simulink model "FinalVersion+AdaptiveSpeedModulation"  (R2024b)
settings: Solver=FixedStepAuto  StartTime=0.0  StopTime=inf  FixedStep=0.001  RelTol=1e-3  EnableMultiTasking=on
libraries: dspnetwork x7
settings Model: xpc_rtwmakecfg_data=_xpcnblib__xpcetherlib__xpcether8255xlib__xpcetherGbElib__xpciplib_  Creator=rudol  LastModifiedBy=Sanjay
settings SolverCC: AlgebraicLoopSolver=TrustRegion
settings DataIOCC: LimitDataPoints=on  SaveFormat=Array  ReturnWorkspaceOutputs=off
settings OptimizationCC: ReuseModelBlockBuffer=off  LifeSpan=inf
settings DebuggingCC: UnconnectedInputMsg=warning  UnconnectedOutputMsg=warning  UnconnectedLineMsg=warning  SFUnexpectedBacktrackingDiag=warning  SFNoUnconditionalDefaultTransitionDiag=warning  SFExecutionAtInitializationDiag=none  ArithmeticOperatorsInVariantConditions=warning
settings HardwareCC: ProdBitPerPointer=32  ProdBitPerSizeT=32  ProdBitPerPtrDiffT=32  ProdLargestAtomicFloat=None  ProdIntDivRoundTo=Undefined  ProdEndianess=Unspecified  ProdWordSize=32  ProdHWDeviceType=32-bit Generic
settings ModelReferenceCC: PropagateSignalLabelsOutOfModel=off
settings SFSimCC: SimUseLocalCustomCode=off  CustomCodeUndefinedFunction=UseInterfaceOnly
settings RTWCC: RTWUseLocalCustomCode=off  GPUComputeCapability=3.5
settings CodeAppCC: StateflowObjectComments=on
settings GRTTargetCC: TargetLangStandard=C89/C90 (ANSI)
settings ConfigComp: CovMetricSettings=dw  CovSaveCumulativeToWorkspaceVar=on  CovSaveSingleToWorkspaceVar=on  CovExternalEMLEnable=off

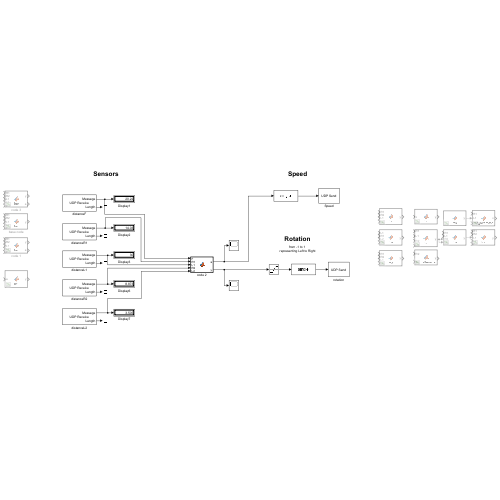
[thumbnail: Simulink's stored preview of the top-level diagram]
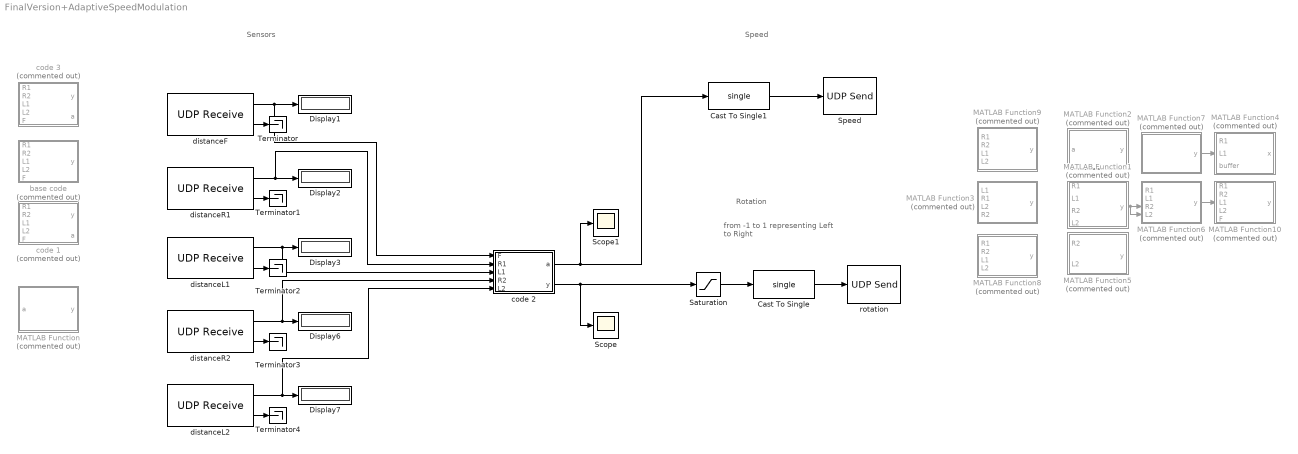
== system FinalVersion+AdaptiveSpeedModulation ==
  note: Sensors
  note: from -1 to 1
      | representing Left to Right
  note: Speed
  note: Rotation
  Cast To Single : DataTypeConversion  OutDataTypeStr=single  SaturateOnIntegerOverflow=off  RndMeth=Floor
  Cast To Single1 : DataTypeConversion  OutDataTypeStr=single  SaturateOnIntegerOverflow=off  RndMeth=Floor
  Display{1..3,6..7} (5 alike) : Display
  MATLAB Function : MATLAB Function  Commented=on  TreatAsAtomicUnit=on
  MATLAB Function1 : MATLAB Function  Commented=on  TreatAsAtomicUnit=on
  MATLAB Function10 : MATLAB Function  Commented=on  TreatAsAtomicUnit=on
  MATLAB Function2 : MATLAB Function  Commented=on  TreatAsAtomicUnit=on
  MATLAB Function3 : MATLAB Function  Commented=on  TreatAsAtomicUnit=on
  MATLAB Function4 : MATLAB Function  Commented=on  TreatAsAtomicUnit=on
  MATLAB Function5 : MATLAB Function  Commented=on  TreatAsAtomicUnit=on
  MATLAB Function6 : MATLAB Function  Commented=on  TreatAsAtomicUnit=on
  MATLAB Function7 : MATLAB Function  Commented=on  TreatAsAtomicUnit=on
  MATLAB Function8 : MATLAB Function  Commented=on  TreatAsAtomicUnit=on
  MATLAB Function9 : MATLAB Function  Commented=on  TreatAsAtomicUnit=on
  Saturation : Saturate  UpperLimit=1  LowerLimit=-1
  Scope : Scope
  Scope1 : Scope
  Speed : dspnetwork/UDP Send  remoteURL='127.0.0.1'  remotePort=55501  localURL='0.0.0.0'  localPortSource=Automatically determine  localPort=-1  sendBufferSize=8192  sampletime=-1  blockPlatform=[]  separateLengthPort=0
  Terminator{,1..4} (5 alike) : Terminator
  base code : MATLAB Function  Commented=on  TreatAsAtomicUnit=on
  code 1 : MATLAB Function  Commented=on  TreatAsAtomicUnit=on
  code 2 : MATLAB Function  TreatAsAtomicUnit=on
  code 3 : MATLAB Function  Commented=on  TreatAsAtomicUnit=on
  distanceF : dspnetwork/UDP Receive  localURL='0.0.0.0'  localPort=10  remoteURL='0.0.0.0'  remotePort=-1  recvBufferSize=8192  dims=1  signalDatatype=single  isComplex=off  isVarSize=off  showBlockingTime=off  blockingTime=0  sampletime=0.001  blockPlatform=[]
  distanceL1 : dspnetwork/UDP Receive  localURL='0.0.0.0'  localPort=12  remoteURL='0.0.0.0'  remotePort=-1  recvBufferSize=8192  dims=1  signalDatatype=single  isComplex=off  isVarSize=off  showBlockingTime=off  blockingTime=0  sampletime=0.001  blockPlatform=[]
  distanceL2 : dspnetwork/UDP Receive  localURL='0.0.0.0'  localPort=14  remoteURL='0.0.0.0'  remotePort=-1  recvBufferSize=8192  dims=1  signalDatatype=single  isComplex=off  isVarSize=off  showBlockingTime=off  blockingTime=0  sampletime=0.001  blockPlatform=[]
  distanceR1 : dspnetwork/UDP Receive  localURL='0.0.0.0'  localPort=11  remoteURL='0.0.0.0'  remotePort=-1  recvBufferSize=8192  dims=1  signalDatatype=single  isComplex=off  isVarSize=off  showBlockingTime=off  blockingTime=0  sampletime=0.001  blockPlatform=[]
  distanceR2 : dspnetwork/UDP Receive  localURL='0.0.0.0'  localPort=13  remoteURL='0.0.0.0'  remotePort=-1  recvBufferSize=8192  dims=1  signalDatatype=single  isComplex=off  isVarSize=off  showBlockingTime=off  blockingTime=0  sampletime=0.001  blockPlatform=[]
  rotation : dspnetwork/UDP Send  remoteURL='127.0.0.1'  remotePort=55000  localURL='0.0.0.0'  localPortSource=Automatically determine  localPort=-1  sendBufferSize=8192  sampletime=-1  blockPlatform=[]  separateLengthPort=0
  wires:
  distanceL1/1 -> Display3/1, code 2/3(L1)
  distanceR1/1 -> code 2/2(R1), Display2/1
  distanceR2/1 -> Display6/1, code 2/4(R2)
  distanceL2/1 -> code 2/5(L2), Display7/1
  Cast To Single/1 -> rotation/1
  distanceF/1 -> Display1/1, code 2/1(F)
  distanceF/2 -> Terminator/1
  distanceR1/2 -> Terminator1/1
  distanceL1/2 -> Terminator2/1
  distanceR2/2 -> Terminator3/1
  distanceL2/2 -> Terminator4/1
  Saturation/1 -> Cast To Single/1
  Cast To Single1/1 -> Speed/1
  code 2/1(a) -> Scope1/1, Cast To Single1/1
  MATLAB Function7/1(y) -> MATLAB Function4/2(L1)
  MATLAB Function1/1(y) -> MATLAB Function6/4(L2), MATLAB Function6/3(R2)
  MATLAB Function6/1(y) -> MATLAB Function10/3(L1)
  code 2/2(y) -> Scope/1, Saturation/1

== matlab function FinalVersion+AdaptiveSpeedModulation/MATLAB Function10 ==
  data: R1 input; y output; R2 input; L1 input; L2 input; F input
function y = fnc(R1, R2, L1, L2, F)
    % Ensure all inputs are of type double to avoid type mismatch
    R1 = double(R1);
    R2 = double(R2);
    L1 = double(L1);
    L2 = double(L2);
    F = double(F);
    y = 0;
    
    % Calculate averages for turning behavior
    avg_RF = (R1 + F) / 2; 
    avg_FL = (F + L1) / 2;   
    avg_R2L2 = (R2 + L2) / 2;  

    % Speed adjustment based on proximity to obstacles
    if R1 < 5 || R2 < 5
        y = -0.7;  
        if R1 < 2.5 || R2 < 2.5
            y = -1;  
        end
    elseif L1 < 5 || L2 < 5
        y = 0.7; 
        if L1 < 5 / 2 || L2 < 5 / 2
            y = 1; 
        end
    end

    % Right turn behavior using front and right-side sensors (smooth turning)
    if avg_RF < 5
        
        y = -1* (5 - avg_RF) ;  
    end

    % Left turn behavior using front and left-side sensors (smooth turning)
    if avg_FL < 5
        
        y =   (5 - avg_FL) ; 
    end

    % Keep the car centered using R2 and L2 (center alignment logic)
    if abs(R2 - L2) > 2.5 
        
        if R2 > L2
            y = y + (R2 - L2) ; 
        elseif L2 > R2
            y = y - (L2 - R2) ; 
        end
    end
    % Additional fine-tuning for smoother operation
    if abs(R2 - L2) < 2.5
        y = y * 0.5;  
    end
end

== matlab function FinalVersion+AdaptiveSpeedModulation/code 1 ==
  data: R1 input; y output; R2 input; L1 input; L2 input; F input; a output
function [y, a] = fnc(R1, R2, L1, L2, F)
    % Ensure all inputs are of type double to avoid type mismatch
    R1 = double(R1);
    R2 = double(R2);
    L1 = double(L1);
    L2 = double(L2);
    F = double(F);
    a = double(F);
    y = 0;  % Steering adjustment
    safe_distance = 5;  % Default safe distance threshold for obstacle avoidance
    
    % Calculate averages for turning behavior
    avg_RF = (R1 + F) / 2;  % Average of Front sensor and Right side sensor
    avg_FL = (F + L1) / 2;  % Average of Front sensor and Left side sensor
    avg_R2L2 = (R2 + L2) / 2;  % Average of Back Right and Back Left sensors (for track center)
    avg_R1L1 = (R1 + L1) / 2;  % Average of Right and Left side sensors (for track center)
     if a < 10
        a = a - (0.2 * F);  % Gradual slowdown based on front sensor proximity
    else
        a = 4 * F;  % Keep a stable speed if the distance is far enough
    end
    
    % Reduce safe distance in the corner (turning condition)
    if abs(avg_RF - avg_FL) > 2  % Corner detected when there is a significant difference in sensor readings
        safe_distance = 3;  % Reduce safe distance during sharp turns
    end
    
    % Speed adjustment based on proximity to obstacles
    if R1 < safe_distance || R2 < safe_distance
        % Slow down if too close to the right side
        y = -5;  % Turn slightly left
        a = 3 * F;  % Reduce speed
        if R1 < safe_distance / 2 || R2 < safe_distance / 2
            y = -10;  % Slow down more if dangerously close to the right side
            a = 2 * F;  % Further reduce speed
        end
    elseif L1 < safe_distance || L2 < safe_distance
        % Speed up if approaching the left side
        y = 5;  % Turn slightly right
        a = 3 * F;  % Increase speed a bit
        if L1 < safe_distance / 2 || L2 < safe_distance / 2
            y = 10;  % Speed up more if dangerously close to the left side
            a = 4 * F;  % Increase speed further
        end
    end
    
    % Smooth turning behavior based on the proximity of the front sensors
    if avg_RF < 3  % Right turn behavior
        y = -5 * (15 - avg_RF) / 15;  % Smooth turning to the right (gradual turn)
        a = 3 * F;  % Maintain speed
    elseif avg_FL < 3  % Left turn behavior
        y = 5 * (15 - avg_FL) / 15;  % Smooth turning to the left (gradual turn)
        a = 3 * F;  % Maintain speed
    end
    
    % Keep the car centered using R2 and L2 (center alignment logic)
    if abs(R2 - L2) > safe_distance / 2  % Check if the car is off-center
        % Apply dynamic steering based on how far off-center the car is
        if R2 > L2
            y = y + 5 * (R2 - L2) / safe_distance;  % Turn left to bring the car back to the center
        elseif L2 > R2
            y = y - 5 * (L2 - R2) / safe_distance;  % Turn right to bring the car back to the center
        end
    end
    
    % % Keep the car centered using R1 and L1 (center alignment logic)
    % if abs(R1 - L1) > safe_distance / 2  % Check if the car is off-center
    %     % Apply dynamic steering based on how far off-center the car is
    %     if R1 > L1
    %         y = y + 5 * (R1 - L1) / safe_distance;  % Turn left to bring the car back to the center
    %     elseif L1 > R1
    %         y = y - 5 * (L1 - R1) / safe_distance;  % Turn right to bring the car back to the center
    %     end
    % end
    
    % Smooth out steering behavior when the rear sensors are close
    if abs(R2 - L2) < safe_distance / 3
        y = y * 0.5;  % Reduce steering to make it smoother when the car is near the center
    end
    
    % High-speed cornering logic (when speed is high and sensors indicate a turn)
    if F > 50 && (avg_RF < safe_distance || avg_FL < safe_distance)
        % Increase turn speed and make it sharper
        if avg_RF < avg_FL
            y = -20;  % Turn right aggressively during sharp turn
            a = 6 * F;  % Maintain higher speed for sharp turn
        else
            y = 20;  % Turn left aggressively during sharp turn
            a = 6 * F;  % Maintain higher speed for sharp turn
        end
    end
    
    % Return the computed steering and acceleration values
end

== matlab function FinalVersion+AdaptiveSpeedModulation/base code ==
  data: R1 input; y output; R2 input; L1 input; L2 input; F input
function y = fnc(R1, R2, L1, L2, F)
    % Ensure all inputs are of type double to avoid type mismatch
    R1 = double(R1);
    R2 = double(R2);
    L1 = double(L1);
    L2 = double(L2);
    F = double(F);
    
    y = 0;
    safe_distance = 5;

    % Calculate averages for turning behavior
    avg_RF = (R1 + F) / 2;  % Average of Front sensor and Right side sensor
    avg_FL = (F + L1) / 2;   % Average of Front sensor and Left side sensor
    avg_R2L2 = (R2 + L2) / 2;  % Average of Back Right and Back Left sensors (for track center)

    % Speed adjustment based on proximity to obstacles
    if R1 < safe_distance || R2 < safe_distance
        y = -10;  % Slow down if too close to the right side
        if R1 < safe_distance / 2 || R2 < safe_distance / 2
            y = -15;  % Slow down more if dangerously close to the right side
        end
    elseif L1 < safe_distance || L2 < safe_distance
        y = 10;  % Speed up if approaching left side
        if L1 < safe_distance / 2 || L2 < safe_distance / 2
            y = 15;  % Speed up more if dangerously close to the left side
        end
    end

    % High-speed turning decision (based on front sensors)
    if (R1 < safe_distance || R2 < safe_distance) && (L1 < safe_distance || L2 < safe_distance)
        if min(R1, R2) > min(L1, L2)
            y = 10;  % Likely turning right, increase right steering
        else
            y = -10;  % Likely turning left, increase left steering
        end
    end

    % Right turn behavior using front and right-side sensors (smooth turning)
    if avg_RF < safe_distance
        % Smooth turning to the right (gradual turn)
        y = -5 * (safe_distance - avg_RF) / safe_distance;  % Adjust turning intensity based on proximity
    end

    % Left turn behavior using front and left-side sensors (smooth turning)
    if avg_FL < safe_distance
        % Smooth turning to the left (gradual turn)
        y = 5 * (safe_distance - avg_FL) / safe_distance;  % Adjust turning intensity based on proximity
    end

    % Keep the car centered using R2 and L2 (center alignment logic)
    if abs(R2 - L2) > safe_distance / 2  % Check if car is off-center
        % Apply a dynamic steering based on how far off-center the car is
        if R2 > L2
            y = y + 5 * (R2 - L2) / safe_distance;  % Turn left to bring the car back to the center
        elseif L2 > R2
            y = y - 5 * (L2 - R2) / safe_distance;  % Turn right to bring the car back to the center
        end
    end

    % Additional fine-tuning for smoother operation
    % If the difference between rear sensors is small, don't apply harsh steering
    if abs(R2 - L2) < safe_distance / 3
        y = y * 0.5;  % Reduce steering to make it smoother when the car is near center
    end
end

== matlab function FinalVersion+AdaptiveSpeedModulation/code 3 ==
  data: R1 input; y output; R2 input; L1 input; L2 input; F input; a output
function [y,a] = fnc(R1, R2, L1, L2, F)
    % Ensure all inputs are of type double to avoid type mismatch
    R1 = double(R1);
    R2 = double(R2);
    L1 = double(L1);
    L2 = double(L2);
    F = double(F);
    a=double(F);
    y = 0;
    safe_distance = 5;
    
    % Calculate averages for turning behavior
    avg_RF = (R1 + F) / 2; % Average of Front sensor and Right side sensor
    avg_FL = (F + L1) / 2; % Average of Front sensor and Left side sensor
    avg_R2L2 = (R2 + L2) / 2; % Average of Back Right and Back Left sensors (for track center)
    avg_R1L1 = (R1 + L1) / 2; % Average of Right and Left side sensors (for track center)
     if a < 10
        a = a -(0.2* F);  
    else
        a = 4*F;  
    end
    
    % Speed adjustment based on proximity to obstacles
    if R1 < safe_distance || R2 < safe_distance
        y = -10; % Slow down if too close to the right side
        a=4*F;
        if R1 < safe_distance / 2 || R2 < safe_distance / 2
            y = -15; % Slow down more if dangerously close to the right side
            a=3.5*F;
        end
    elseif L1 < safe_distance || L2 < safe_distance
        y = 10; % Speed up if approaching left side
        a=4*F;
        if L1 < safe_distance / 2 || L2 < safe_distance / 2
            y = 15; % Speed up more if dangerously close to the left side
            a=3.5*F;
        end
    end
    
    % High-speed turning decision (based on front sensors)
    if (R1 < safe_distance || R2 < safe_distance) && (L1 < safe_distance || L2 < safe_distance)
        if min(R1, R2) > min(L1, L2)
            y = 10; % Likely turning right, increase right steering
            a=4*F;
        else
            y = -10; % Likely turning left, increase left steering
            a=6*F;
        end
    end
    
    % Right turn behavior using front and right-side sensors (smooth turning)
    if avg_RF < 3
        % Smooth turning to the right (gradual turn)
        y = -5 * (15 - avg_RF) / 15; % Adjust turning intensity based on proximity
        a=4.5*F;
    end
    
    % Left turn behavior using front and left-side sensors (smooth turning)
    if avg_FL < 3
        % Smooth turning to the left (gradual turn)
        y = 5 * (15 - avg_FL) / 15; % Adjust turning intensity based on proximity
        a=4.5*F;
    end
    
    % Keep the car centered using R2 and L2 (center alignment logic)
    if abs(R2 - L2) > safe_distance / 2
        % Check if car is off-center
        % Apply a dynamic steering based on how far off-center the car is
        if R2 > L2
            y = y + 5 * (R2 - L2) / safe_distance; % Turn left to bring the car back to the center
        elseif L2 > R2
            y = y - 5 * (L2 - R2) / safe_distance; % Turn right to bring the car back to the center
        end
    end
    
    % Keep the car centered using R1 and L1 (center alignment logic)
    if abs(R1 - L1) > safe_distance / 2
        % Check if car is off-center
        % Apply a dynamic steering based on how far off-center the car is
        if R1 > L1
            y = y + 5 * (R1 - L1) / safe_distance; % Turn left to bring the car back to the center
        elseif L1 > R1
            y = y - 5 * (L1 - R1) / safe_distance; % Turn right to bring the car back to the center
        end
    end
    
    % Additional fine-tuning for smoother operation
    % If the difference between rear sensors is small, don't apply harsh steering
    if abs(R2 - L2) < safe_distance / 3
        y = y * 0.5; % Reduce steering to make it smoother when the car is near center
    end
    
    % High-speed cornering logic
    if F > 50 && (avg_RF < safe_distance || avg_FL < safe_distance)
        if avg_RF < avg_FL
            y = -15; % Turn right sharply
            a=4*F;
        else
            y = 15; % Turn left sharply
            a=4*F;
        end
    end
end

== matlab function FinalVersion+AdaptiveSpeedModulation/code 2 ==
  data: F input; a output; R1 input; L1 input; y output; R2 input; L2 input
function [a, y] = fnc(F,R1, L1, R2, L2)
    R1 = double(R1);
    R2 = double(R2);
    L1 = double(L1);
    L2 = double(L2);
    F = double(F);
    a = double(F);
    y = 0;  
     
    avg_RF = (R1 + F) / 2;  
    avg_FL = (F + L1) / 2;  
    avg_R2L2 = (R2 + L2) / 2;  % this function not used in logic 
    avg_R1L1 = (R1 + L1) / 2;  % this function not used in logic 
    
    if a < 10        
        a = a - (0.2 * F);  % I reduced the car speed gradually based on front sensor proximity
    else
        a = 4.5* F; 
   end    
    
   %buffer zone =5;
    
   if R1 < 5 || R2 < 5               
        y = -0.5;   % turn left slightly based on if condition
        a = 3 * F; 
       
        %buffer zone =5;
        %(buffer zone/2)=2.5;
        if R1 < 2.5 || R2 < 2.5
            y = -1;  % it will turn left suddenly
            a = 4 * F;  
        end
        
        %buffer zone =5;
    elseif L1 < 5 || L2 < 5
        
        y = 0.5;  % Turn slightly right
        a = 3 * F;  
        
        %buffer zone =5;
        %(buffer zone/2)=2.5;
        if L1 < 2.5|| L2 < 2.5
            y = 1;  % it will rurn right suddenly
            a = 4 * F; 
        end
    end
    
    if avg_RF < 3 
        y = -5 * (15 - avg_RF) / 15;  %gradual turn
        a = 3 * F;  
    elseif avg_FL < 3 
        y = 5 * (15 - avg_FL) / 15;  % gradual turn
        a = 3 * F;  
    end

    %buffer zone =3; (buffer zone / 2)=1.5;
    if abs(R2 - L2) >1.5  % Check if the car is off-center  
        
        if R2 > L2
            y = y + 5 * (R2 - L2) / 3;  % Turn left to bring the car back to the center
        elseif L2 > R2
            y = y - 5 * (L2 - R2) / 3;  % Turn right to bring the car back to the center
        end
    end
    
    %buffer zone =3; (buffer zone / 2)=1.5;
    if abs(R1 - L1) > 1.5  % Check if the car is off-center
        if R1 > L1
            y = y + 5 * (R1 - L1) / 3;  % Turn left to bring the car back to the center
        elseif L1 > R1
            y = y - 5 * (L1 - R1) / 3;  % Turn right to bring the car back to the center
        end
    end
    
   %buffer zone =5;
    if abs(R2 - L2) < 5 / 3
        y = y * 0.5;  % Reduce steering to make it smoother when the car is near the center
    end
    
    %buffer zone = 5;
    if F > 50 && (avg_RF < 5 || avg_FL < 5)   %  when speed is high and sensors indicate a turn
        if avg_RF < avg_FL
            y = -15;  % Turn right sharply
            a = 4 * F;  
        else
            y = 15;  % Turn left sharply
            a = 4 * F;  
        end
    end
end

== matlab function FinalVersion+AdaptiveSpeedModulation/MATLAB Function1 ==
  data: R1 input; L1 input; R2 input; y output; L2 input
function y = fcn(R1, L1,R2,L2)
  Kp = 1.5;
    left_distance = (L1 + L2) / 2;
    right_distance = (R1 + R2) / 2;
    error = left_distance - right_distance;
    y = -Kp * error;
    safe_distance = 20; 
    max_steering_angle = 30; 

    if R1 < safe_distance
        right_adjustment = max_steering_angle * (safe_distance - R1) / safe_distance;
        y = y + right_adjustment;
    end
     
    if L1 < safe_distance
        left_adjustment = max_steering_angle * (safe_distance - L1) / safe_distance;
        y = y - left_adjustment;
    end
    if R2 < safe_distance
        right_adjustment = max_steering_angle * (safe_distance - R2) / safe_distance;
        y = y + right_adjustment * 0.5;
    end

    if L2 < safe_distance
        left_adjustment = max_steering_angle * (safe_distance - L2) / safe_distance;
        y = y - left_adjustment * 0.5;
    end
 y = max(min(y, max_steering_angle), -max_steering_angle);

   
end

== matlab function FinalVersion+AdaptiveSpeedModulation/MATLAB Function ==
  data: a input; y output
function y = fcn(a)    
    
    if a < 10
        a = a -(0.2* a);  
    else
        a = a + (4.5* a);  
    end
  
y=a;
end



  % a: current speed
    % curvature: turn's curvature (higher value means tighter turn)

    %if curvature > 0.5
        % Tight turn, reduce speed
        %a = a - (0.2 * a);
    %elseif curvature < -0.5
        % Tight turn, reduce speed
       % a = a - (0.2 * a);
   % else
        % Smooth turn or straight path, maintain or increase speed
       % a = a + (0.1 * a);
    %end

== matlab function FinalVersion+AdaptiveSpeedModulation/MATLAB Function2 ==
  data: a input; y output
function y = fcn(a)
    
    a = single(a);  
    max_speed = single(50);         
    close_distance = single(20);    
    speed_increment = single(5);    
    distance = single(100) - a;     
    if distance > close_distance
        a = a + speed_increment;  
        if a > max_speed
            a = max_speed;       
        end
    else
        a = a;  
    end
    y = a; 
end

== matlab function FinalVersion+AdaptiveSpeedModulation/MATLAB Function3 ==
  data: L1 input; y output; R1 input; L2 input; R2 input
function y = fcn(L1, R1, L2, R2)
    
    Kp = 1.5; 
    safe_distance = 20; 
    max_steering_angle = 30; 
    target_range = 4; 
    

    left_distance = (L1 + L2) / 2;
    right_distance = (R1 + R2) / 2;
    error = left_distance - right_distance;
    
  
    y = -Kp * error;

    
    if R1 < safe_distance
        right_adjustment = max_steering_angle * (safe_distance - R1) / safe_distance;
        y = y + right_adjustment;
    end
    if R2 < safe_distance
        right_adjustment = max_steering_angle * (safe_distance - R2) / safe_distance;
        y = y + right_adjustment * 0.5;
    end

    if L1 < safe_distance
        left_adjustment = max_steering_angle * (safe_distance - L1) / safe_distance;
        y = y - left_adjustment;
    end
    if L2 < safe_distance
        left_adjustment = max_steering_angle * (safe_distance - L2) / safe_distance;
        y = y - left_adjustment * 0.5;
    end

   
    y = max(min(y, max_steering_angle), -max_steering_angle);

   
    y = y / max_steering_angle * target_range;

   
    y = max(min(y, target_range), -target_range);
end

== matlab function FinalVersion+AdaptiveSpeedModulation/MATLAB Function4 ==
  data: R1 input; x output; L1 input; buffer input
function x = fcn_alternate(R1, L1, buffer)
    c_factor = 15;
    
    % Calculate the mean of R1 and L1
    m = (R1 + L1) / 2;
    
    % Determine deviation from the mean
    deviation = 0;  % Initialize
    if R1 - m > buffer
        deviation = double(R1 - m);
    elseif L1 - m > buffer
        deviation = double(-(L1 - m));
    end
    
    % Compute output based on deviation
    x = double(deviation / c_factor);
end

== matlab function FinalVersion+AdaptiveSpeedModulation/MATLAB Function5 ==
  data: R2 input; y output; L2 input
function y = fcn_alternate(R2, L2)
    c_factor = 22;  
    buffer = 0.2;  

    % Calculate the difference between R2 and L2
    dist = R2 - L2;

    % Initialize adjustment variable
    n = 0;

    % Logic for determining adjustment
    if abs(dist) > buffer
        n = double(dist); % Deviation based on distance difference
    elseif min(R2, L2) < 0.5
        n =double (-(min(R2, L2))); % React to proximity
    end

    % Compute output
    y = n / c_factor;
end

== matlab function FinalVersion+AdaptiveSpeedModulation/MATLAB Function6 ==
  data: R1 input; y output; L1 input; R2 input; L2 input
function y = fcn(R1, L1, R2, L2)
    % Constants
    c_factor1 = 15;  
    c_factor2 = 22;  
    buffer1 = 0.2;  
    buffer2 = 0.2;  

    % Part 1: R1 and L1 Logic
    m = (R1 + L1) / 2; % Calculate the mean
    deviation1 = 0; % Initialize deviation for R1 and L1
    if R1 - m > buffer1
        deviation1 = double(R1 - m);
    elseif L1 - m > buffer1
        deviation1 = double(-(L1 - m));
    end
    output1 = double(deviation1 / c_factor1); % Output from R1 and L1 logic

    % Part 2: R2 and L2 Logic
    dist = R2 - L2; % Calculate difference between R2 and L2
    deviation2 = 0; % Initialize deviation for R2 and L2
    if abs(dist) > buffer2
        deviation2 = double(dist); % Deviation based on distance
    elseif min(R2, L2) < 0.5
        deviation2 = double(-(min(R2, L2))); % React to proximity
    end
    output2 = double(deviation2 / c_factor2); % Output from R2 and L2 logic

    % Combine the outputs (logic can be adjusted as needed)
    y = output1 + output2; % Final combined output
end

== matlab function FinalVersion+AdaptiveSpeedModulation/MATLAB Function7 ==
  data: y output
function y = fcn()

y = u;

== matlab function FinalVersion+AdaptiveSpeedModulation/MATLAB Function8 ==
  data: R1 input; y output; R2 input; L1 input; L2 input
function y = fnc(R1, R2, L1, L2)
    % Inputs:
    % R1: Right-top sensor reading
    % R2: Right-rear sensor reading
    % L1: Left-top sensor reading
    % L2: Left-rear sensor reading

    % Initialize steering angle (0 means no adjustment)
    y = 0;

    % Set safe distance threshold (hardcoded for simplicity)
    safe_distance = 5; % in meters, adjust as needed

    % Check for proximity to the right-side wall
    if R1 < safe_distance || R2 < safe_distance
        % Wall detected on the right, steer left
        y = -15; % Adjust this value for sharper turns
    end

    % Check for proximity to the left-side wall
    if L1 < safe_distance || L2 < safe_distance
        % Wall detected on the left, steer right
        y = 15; % Adjust this value for sharper turns
    end

    % Handle cases where both sides are close to walls
    if (R1 < safe_distance || R2 < safe_distance) && (L1 < safe_distance || L2 < safe_distance)
        % Prioritize steering to the side with more space
        if min(R1, R2) > min(L1, L2)
            y = 15; % Steer right
        else
            y = -15; % Steer left
        end
    end
end

== matlab function FinalVersion+AdaptiveSpeedModulation/MATLAB Function9 ==
  data: R1 input; R2 input; L1 input; y output; L2 input

function y = fnc(R1, R2, L1, L2)
    y = 0;
    safe_distance = 5;

    if R1 < 5 || R2 < 5

        y = -0.5;

    elseif R1 < 2.5 || R2 < 2.5
            y = -1; 
    end


    if L1 < 5|| L2 < 5

        y = 0.5; 


    elseif L1 < 2.5 || L2 <2.5
            y = 1;
    end


    if (R1 < safe_distance || R2 < safe_distance) && (L1 < safe_distance || L2 < safe_distance)

        if min(R1, R2) > min(L1, L2)
            y = 0.5; 
        else
            y = -0.5; 
        end
    end
